simulink model "level3_MMC"  (Simulink 9.0)
settings: Solver=VariableStepAuto  StartTime=0.0  StopTime=10.0  RelTol=1e-3
libraries: powerlib x60
settings Model: Creator=lenovo  LastModifiedBy=lenovo
settings DataIOCC: SaveFormat=Dataset
settings OptimizationCC: LifeSpan=auto
settings DebuggingCC: UnderspecifiedInitializationDetection=Simplified  MergeDetectMultiDrivingBlocksExec=error  SFUnexpectedBacktrackingDiag=error  SFNoUnconditionalDefaultTransitionDiag=error  SFExecutionAtInitializationDiag=warning
settings HardwareCC: ProdBitPerPointer=64  ProdBitPerSizeT=64  ProdBitPerPtrDiffT=64  ProdLargestAtomicFloat=Float  ProdIntDivRoundTo=Zero  ProdEndianess=LittleEndian  ProdWordSize=64  ProdHWDeviceType=Intel->x86-64 (Windows64)
settings ModelReferenceCC: PropagateSignalLabelsOutOfModel=on
settings CodeAppCC: StateflowObjectComments=off
settings GRTTargetCC: TargetLangStandard=C99 (ISO)
settings ConfigComp: CovMetricSettings=dwe  CovHtmlReporting=off  CovSaveCumulativeToWorkspaceVar=off  CovSaveSingleToWorkspaceVar=off  CovExternalEMLEnable=on

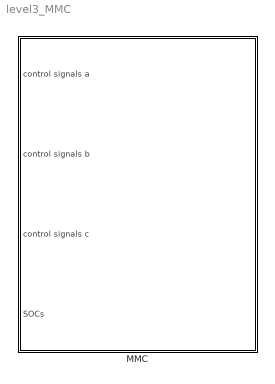
== system level3_MMC ==
  MMC : Subsystem

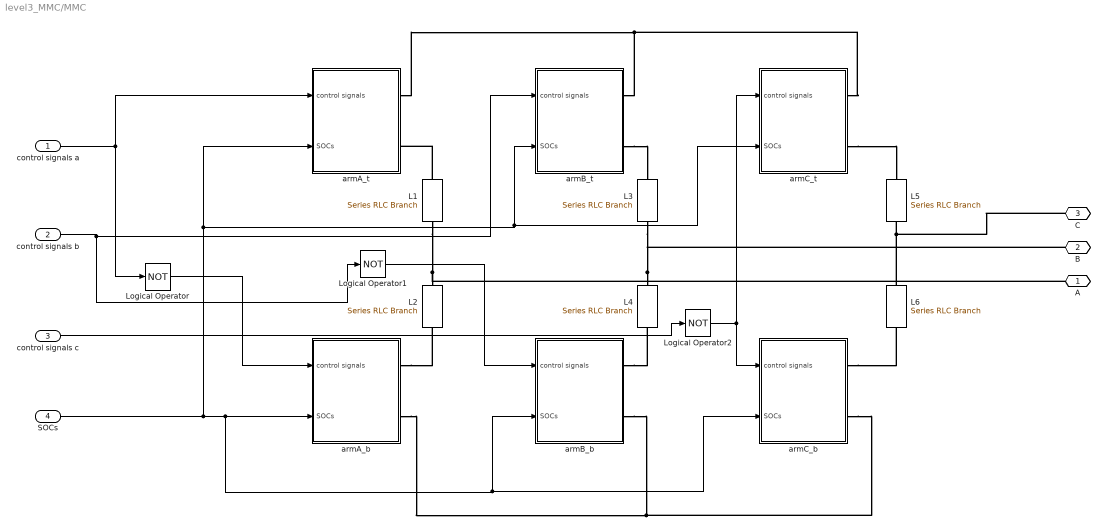
== system level3_MMC/MMC ==
  control signals a : Inport
  control signals b : Inport  Port=2
  control signals c : Inport  Port=3
  SOCs : Inport  Port=4
  L{1..6} (6 alike) : powerlib/Elements/Series RLC Branch  LConnTagsString=__new0  RConnTagsString=__new0  BranchType=L  Resistance=0  Inductance=50e-6  SetiL0=off  InitialCurrent=0  Capacitance=0  Setx0=off  InitialVoltage=0  Measurements=None
  Logical Operator : Logic  Operator=NOT  AllPortsSameDT=off  OutDataTypeStr=boolean
  Logical Operator1 : Logic  Operator=NOT  AllPortsSameDT=off  OutDataTypeStr=boolean
  Logical Operator2 : Logic  Operator=NOT  AllPortsSameDT=off  OutDataTypeStr=boolean
  armA_b : Subsystem
  armA_t : Subsystem
  armB_b : Subsystem
  armB_t : Subsystem
  armC_b : Subsystem
  armC_t : Subsystem
  A : PMIOPort  Port=1  Side=Right
  B : PMIOPort  Port=2  Side=Right
  C : PMIOPort  Port=3  Side=Right
  wires:
  SOCs/1 -> armA_b/2(SOCs), armC_b/2(SOCs), armB_b/2(SOCs), armA_t/2(SOCs), armC_t/2(SOCs), armB_t/2(SOCs)
  Logical Operator1/1 -> armB_b/1(control signals)
  control signals b/1 -> armB_t/1(control signals), Logical Operator1/1
  Logical Operator/1 -> armA_b/1(control signals)
  control signals a/1 -> armA_t/1(control signals), Logical Operator/1
  Logical Operator2/1 -> armC_b/1(control signals), armC_t/1(control signals)
  control signals c/1 -> Logical Operator2/1
  connections:
  L6/LConn1 -- C/RConn1 -- L5/RConn1
  L1/LConn1 -- armA_t/RConn2
  armC_t/RConn2 -- L5/LConn1
  armC_b/RConn1 -- L6/RConn1
  armB_t/RConn2 -- L3/LConn1
  armB_b/RConn1 -- L4/RConn1
  armA_b/RConn1 -- L2/RConn1
  L4/LConn1 -- L3/RConn1 -- B/RConn1
  L1/RConn1 -- L2/LConn1 -- A/RConn1
  armA_b/RConn2 -- armC_b/RConn2 -- armB_b/RConn2
  armA_t/RConn1 -- armC_t/RConn1 -- armB_t/RConn1

== system level3_MMC/MMC/armA_b ==
  control signals : Inport
  SOCs : Inport  Port=2
  SubModule1 : Subsystem
  SubModule2 : Subsystem
  SubModule3 : Subsystem
  Conn1 : PMIOPort  Port=1  Side=Right
  Conn2 : PMIOPort  Port=2  Side=Right
  wires:
  control signals/1 -> SubModule3/1(control signal), SubModule2/1(control signal), SubModule1/1(control signal)
  SOCs/1 -> SubModule3/2(SOC), SubModule2/2(SOC), SubModule1/2(SOC)
  connections:
  SubModule1/RConn2 -- SubModule2/RConn1
  SubModule1/RConn1 -- Conn1/RConn1
  Conn2/RConn1 -- SubModule3/RConn2
  SubModule2/RConn2 -- SubModule3/RConn1

== system level3_MMC/MMC/armA_t ==
  control signals : Inport
  SOCs : Inport  Port=2
  SubModule1 : Subsystem
  SubModule2 : Subsystem
  SubModule3 : Subsystem
  Conn1 : PMIOPort  Port=1  Side=Right
  Conn2 : PMIOPort  Port=2  Side=Right
  wires:
  control signals/1 -> SubModule3/1(control signal), SubModule2/1(control signal), SubModule1/1(control signal)
  SOCs/1 -> SubModule3/2(SOC), SubModule2/2(SOC), SubModule1/2(SOC)
  connections:
  SubModule1/RConn2 -- SubModule2/RConn1
  SubModule1/RConn1 -- Conn1/RConn1
  Conn2/RConn1 -- SubModule3/RConn2
  SubModule2/RConn2 -- SubModule3/RConn1

== system level3_MMC/MMC/armB_b ==
  control signals : Inport
  SOCs : Inport  Port=2
  SubModule1 : Subsystem
  SubModule2 : Subsystem
  SubModule3 : Subsystem
  Conn1 : PMIOPort  Port=1  Side=Right
  Conn2 : PMIOPort  Port=2  Side=Right
  wires:
  control signals/1 -> SubModule3/1(control signal), SubModule2/1(control signal), SubModule1/1(control signal)
  SOCs/1 -> SubModule3/2(SOC), SubModule2/2(SOC), SubModule1/2(SOC)
  connections:
  SubModule1/RConn2 -- SubModule2/RConn1
  SubModule1/RConn1 -- Conn1/RConn1
  Conn2/RConn1 -- SubModule3/RConn2
  SubModule2/RConn2 -- SubModule3/RConn1

== system level3_MMC/MMC/armB_t ==
  control signals : Inport
  SOCs : Inport  Port=2
  SubModule1 : Subsystem
  SubModule2 : Subsystem
  SubModule3 : Subsystem
  Conn1 : PMIOPort  Port=1  Side=Right
  Conn2 : PMIOPort  Port=2  Side=Right
  wires:
  control signals/1 -> SubModule3/1(control signal), SubModule2/1(control signal), SubModule1/1(control signal)
  SOCs/1 -> SubModule3/2(SOC), SubModule2/2(SOC), SubModule1/2(SOC)
  connections:
  SubModule1/RConn2 -- SubModule2/RConn1
  SubModule1/RConn1 -- Conn1/RConn1
  Conn2/RConn1 -- SubModule3/RConn2
  SubModule2/RConn2 -- SubModule3/RConn1

== system level3_MMC/MMC/armC_b ==
  control signals : Inport
  SOCs : Inport  Port=2
  SubModule1 : Subsystem
  SubModule2 : Subsystem
  SubModule3 : Subsystem
  Conn1 : PMIOPort  Port=1  Side=Right
  Conn2 : PMIOPort  Port=2  Side=Right
  wires:
  control signals/1 -> SubModule3/1(control signal), SubModule2/1(control signal), SubModule1/1(control signal)
  SOCs/1 -> SubModule3/2(SOC), SubModule2/2(SOC), SubModule1/2(SOC)
  connections:
  SubModule1/RConn2 -- SubModule2/RConn1
  SubModule1/RConn1 -- Conn1/RConn1
  Conn2/RConn1 -- SubModule3/RConn2
  SubModule2/RConn2 -- SubModule3/RConn1

== system level3_MMC/MMC/armC_t ==
  control signals : Inport
  SOCs : Inport  Port=2
  SubModule1 : Subsystem
  SubModule2 : Subsystem
  SubModule3 : Subsystem
  Conn1 : PMIOPort  Port=1  Side=Right
  Conn2 : PMIOPort  Port=2  Side=Right
  wires:
  control signals/1 -> SubModule3/1(control signal), SubModule2/1(control signal), SubModule1/1(control signal)
  SOCs/1 -> SubModule3/2(SOC), SubModule2/2(SOC), SubModule1/2(SOC)
  connections:
  SubModule1/RConn2 -- SubModule2/RConn1
  SubModule1/RConn1 -- Conn1/RConn1
  Conn2/RConn1 -- SubModule3/RConn2
  SubModule2/RConn2 -- SubModule3/RConn1

== system level3_MMC/MMC/armA_b/SubModule1 ==
  control signal : Inport
  SOC : Inport  Port=2
  MOSFET : Subsystem
  cell voltage : Subsystem
  P1 : PMIOPort  Tag=PMCPort  Port=1  Side=Right
  P2 : PMIOPort  Tag=PMCPort  Port=2  Side=Right
  wires:
  control signal/1 -> MOSFET/1(control signal)
  cell voltage/1(V) -> MOSFET/2(V)
  SOC/1 -> cell voltage/1(SOC)
  connections:
  P1/RConn1 -- MOSFET/RConn1
  P2/RConn1 -- MOSFET/RConn2

== system level3_MMC/MMC/armA_b/SubModule2 ==
  control signal : Inport
  SOC : Inport  Port=2
  MOSFET : Subsystem
  cell voltage : Subsystem
  P1 : PMIOPort  Tag=PMCPort  Port=1  Side=Right
  P2 : PMIOPort  Tag=PMCPort  Port=2  Side=Right
  wires:
  control signal/1 -> MOSFET/1(control signal)
  cell voltage/1(V) -> MOSFET/2(V)
  SOC/1 -> cell voltage/1(SOC)
  connections:
  P1/RConn1 -- MOSFET/RConn1
  P2/RConn1 -- MOSFET/RConn2

== system level3_MMC/MMC/armA_b/SubModule3 ==
  control signal : Inport
  SOC : Inport  Port=2
  MOSFET : Subsystem
  cell voltage : Subsystem
  P1 : PMIOPort  Tag=PMCPort  Port=1  Side=Right
  P2 : PMIOPort  Tag=PMCPort  Port=2  Side=Right
  wires:
  control signal/1 -> MOSFET/1(control signal)
  cell voltage/1(V) -> MOSFET/2(V)
  SOC/1 -> cell voltage/1(SOC)
  connections:
  P1/RConn1 -- MOSFET/RConn1
  P2/RConn1 -- MOSFET/RConn2

== system level3_MMC/MMC/armA_t/SubModule1 ==
  control signal : Inport
  SOC : Inport  Port=2
  MOSFET : Subsystem
  cell voltage : Subsystem
  P1 : PMIOPort  Tag=PMCPort  Port=1  Side=Right
  P2 : PMIOPort  Tag=PMCPort  Port=2  Side=Right
  wires:
  control signal/1 -> MOSFET/1(control signal)
  cell voltage/1(V) -> MOSFET/2(V)
  SOC/1 -> cell voltage/1(SOC)
  connections:
  P1/RConn1 -- MOSFET/RConn1
  P2/RConn1 -- MOSFET/RConn2

== system level3_MMC/MMC/armA_t/SubModule2 ==
  control signal : Inport
  SOC : Inport  Port=2
  MOSFET : Subsystem
  cell voltage : Subsystem
  P1 : PMIOPort  Tag=PMCPort  Port=1  Side=Right
  P2 : PMIOPort  Tag=PMCPort  Port=2  Side=Right
  wires:
  control signal/1 -> MOSFET/1(control signal)
  cell voltage/1(V) -> MOSFET/2(V)
  SOC/1 -> cell voltage/1(SOC)
  connections:
  P1/RConn1 -- MOSFET/RConn1
  P2/RConn1 -- MOSFET/RConn2

== system level3_MMC/MMC/armA_t/SubModule3 ==
  control signal : Inport
  SOC : Inport  Port=2
  MOSFET : Subsystem
  cell voltage : Subsystem
  P1 : PMIOPort  Tag=PMCPort  Port=1  Side=Right
  P2 : PMIOPort  Tag=PMCPort  Port=2  Side=Right
  wires:
  control signal/1 -> MOSFET/1(control signal)
  cell voltage/1(V) -> MOSFET/2(V)
  SOC/1 -> cell voltage/1(SOC)
  connections:
  P1/RConn1 -- MOSFET/RConn1
  P2/RConn1 -- MOSFET/RConn2

== system level3_MMC/MMC/armB_b/SubModule1 ==
  control signal : Inport
  SOC : Inport  Port=2
  MOSFET : Subsystem
  cell voltage : Subsystem
  P1 : PMIOPort  Tag=PMCPort  Port=1  Side=Right
  P2 : PMIOPort  Tag=PMCPort  Port=2  Side=Right
  wires:
  control signal/1 -> MOSFET/1(control signal)
  cell voltage/1(V) -> MOSFET/2(V)
  SOC/1 -> cell voltage/1(SOC)
  connections:
  P1/RConn1 -- MOSFET/RConn1
  P2/RConn1 -- MOSFET/RConn2

== system level3_MMC/MMC/armB_b/SubModule2 ==
  control signal : Inport
  SOC : Inport  Port=2
  MOSFET : Subsystem
  cell voltage : Subsystem
  P1 : PMIOPort  Tag=PMCPort  Port=1  Side=Right
  P2 : PMIOPort  Tag=PMCPort  Port=2  Side=Right
  wires:
  control signal/1 -> MOSFET/1(control signal)
  cell voltage/1(V) -> MOSFET/2(V)
  SOC/1 -> cell voltage/1(SOC)
  connections:
  P1/RConn1 -- MOSFET/RConn1
  P2/RConn1 -- MOSFET/RConn2

== system level3_MMC/MMC/armB_b/SubModule3 ==
  control signal : Inport
  SOC : Inport  Port=2
  MOSFET : Subsystem
  cell voltage : Subsystem
  P1 : PMIOPort  Tag=PMCPort  Port=1  Side=Right
  P2 : PMIOPort  Tag=PMCPort  Port=2  Side=Right
  wires:
  control signal/1 -> MOSFET/1(control signal)
  cell voltage/1(V) -> MOSFET/2(V)
  SOC/1 -> cell voltage/1(SOC)
  connections:
  P1/RConn1 -- MOSFET/RConn1
  P2/RConn1 -- MOSFET/RConn2

== system level3_MMC/MMC/armB_t/SubModule1 ==
  control signal : Inport
  SOC : Inport  Port=2
  MOSFET : Subsystem
  cell voltage : Subsystem
  P1 : PMIOPort  Tag=PMCPort  Port=1  Side=Right
  P2 : PMIOPort  Tag=PMCPort  Port=2  Side=Right
  wires:
  control signal/1 -> MOSFET/1(control signal)
  cell voltage/1(V) -> MOSFET/2(V)
  SOC/1 -> cell voltage/1(SOC)
  connections:
  P1/RConn1 -- MOSFET/RConn1
  P2/RConn1 -- MOSFET/RConn2

== system level3_MMC/MMC/armB_t/SubModule2 ==
  control signal : Inport
  SOC : Inport  Port=2
  MOSFET : Subsystem
  cell voltage : Subsystem
  P1 : PMIOPort  Tag=PMCPort  Port=1  Side=Right
  P2 : PMIOPort  Tag=PMCPort  Port=2  Side=Right
  wires:
  control signal/1 -> MOSFET/1(control signal)
  cell voltage/1(V) -> MOSFET/2(V)
  SOC/1 -> cell voltage/1(SOC)
  connections:
  P1/RConn1 -- MOSFET/RConn1
  P2/RConn1 -- MOSFET/RConn2

== system level3_MMC/MMC/armB_t/SubModule3 ==
  control signal : Inport
  SOC : Inport  Port=2
  MOSFET : Subsystem
  cell voltage : Subsystem
  P1 : PMIOPort  Tag=PMCPort  Port=1  Side=Right
  P2 : PMIOPort  Tag=PMCPort  Port=2  Side=Right
  wires:
  control signal/1 -> MOSFET/1(control signal)
  cell voltage/1(V) -> MOSFET/2(V)
  SOC/1 -> cell voltage/1(SOC)
  connections:
  P1/RConn1 -- MOSFET/RConn1
  P2/RConn1 -- MOSFET/RConn2

== system level3_MMC/MMC/armC_b/SubModule1 ==
  control signal : Inport
  SOC : Inport  Port=2
  MOSFET : Subsystem
  cell voltage : Subsystem
  P1 : PMIOPort  Tag=PMCPort  Port=1  Side=Right
  P2 : PMIOPort  Tag=PMCPort  Port=2  Side=Right
  wires:
  control signal/1 -> MOSFET/1(control signal)
  cell voltage/1(V) -> MOSFET/2(V)
  SOC/1 -> cell voltage/1(SOC)
  connections:
  P1/RConn1 -- MOSFET/RConn1
  P2/RConn1 -- MOSFET/RConn2

== system level3_MMC/MMC/armC_b/SubModule2 ==
  control signal : Inport
  SOC : Inport  Port=2
  MOSFET : Subsystem
  cell voltage : Subsystem
  P1 : PMIOPort  Tag=PMCPort  Port=1  Side=Right
  P2 : PMIOPort  Tag=PMCPort  Port=2  Side=Right
  wires:
  control signal/1 -> MOSFET/1(control signal)
  cell voltage/1(V) -> MOSFET/2(V)
  SOC/1 -> cell voltage/1(SOC)
  connections:
  P1/RConn1 -- MOSFET/RConn1
  P2/RConn1 -- MOSFET/RConn2

== system level3_MMC/MMC/armC_b/SubModule3 ==
  control signal : Inport
  SOC : Inport  Port=2
  MOSFET : Subsystem
  cell voltage : Subsystem
  P1 : PMIOPort  Tag=PMCPort  Port=1  Side=Right
  P2 : PMIOPort  Tag=PMCPort  Port=2  Side=Right
  wires:
  control signal/1 -> MOSFET/1(control signal)
  cell voltage/1(V) -> MOSFET/2(V)
  SOC/1 -> cell voltage/1(SOC)
  connections:
  P1/RConn1 -- MOSFET/RConn1
  P2/RConn1 -- MOSFET/RConn2

== system level3_MMC/MMC/armC_t/SubModule1 ==
  control signal : Inport
  SOC : Inport  Port=2
  MOSFET : Subsystem
  cell voltage : Subsystem
  P1 : PMIOPort  Tag=PMCPort  Port=1  Side=Right
  P2 : PMIOPort  Tag=PMCPort  Port=2  Side=Right
  wires:
  control signal/1 -> MOSFET/1(control signal)
  cell voltage/1(V) -> MOSFET/2(V)
  SOC/1 -> cell voltage/1(SOC)
  connections:
  P1/RConn1 -- MOSFET/RConn1
  P2/RConn1 -- MOSFET/RConn2

== system level3_MMC/MMC/armC_t/SubModule2 ==
  control signal : Inport
  SOC : Inport  Port=2
  MOSFET : Subsystem
  cell voltage : Subsystem
  P1 : PMIOPort  Tag=PMCPort  Port=1  Side=Right
  P2 : PMIOPort  Tag=PMCPort  Port=2  Side=Right
  wires:
  control signal/1 -> MOSFET/1(control signal)
  cell voltage/1(V) -> MOSFET/2(V)
  SOC/1 -> cell voltage/1(SOC)
  connections:
  P1/RConn1 -- MOSFET/RConn1
  P2/RConn1 -- MOSFET/RConn2

== system level3_MMC/MMC/armC_t/SubModule3 ==
  control signal : Inport
  SOC : Inport  Port=2
  MOSFET : Subsystem
  cell voltage : Subsystem
  P1 : PMIOPort  Tag=PMCPort  Port=1  Side=Right
  P2 : PMIOPort  Tag=PMCPort  Port=2  Side=Right
  wires:
  control signal/1 -> MOSFET/1(control signal)
  cell voltage/1(V) -> MOSFET/2(V)
  SOC/1 -> cell voltage/1(SOC)
  connections:
  P1/RConn1 -- MOSFET/RConn1
  P2/RConn1 -- MOSFET/RConn2

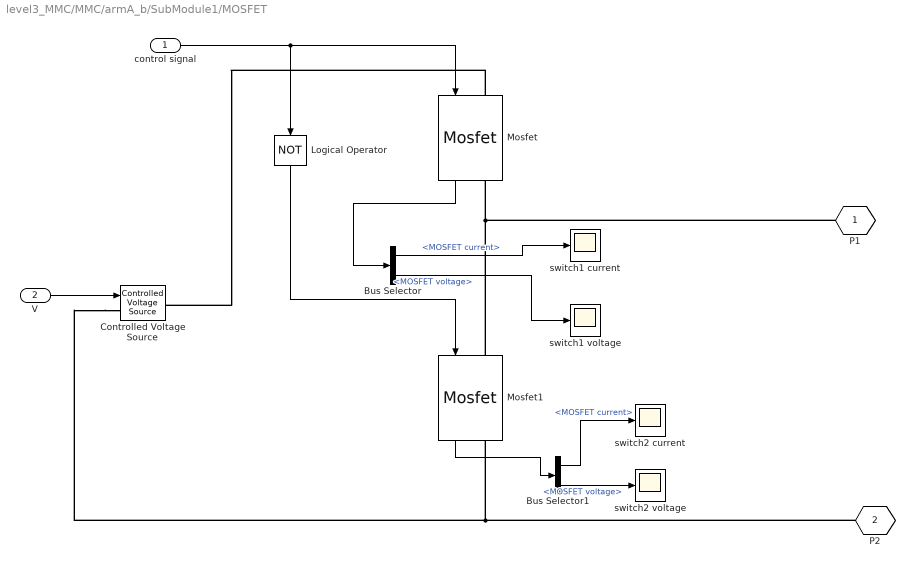
== system level3_MMC/MMC/armA_b/SubModule1/MOSFET ==
  control signal : Inport
  V : Inport  Port=2
  Bus Selector : BusSelector  OutputSignals=MOSFET current,MOSFET voltage
  Bus Selector1 : BusSelector  OutputSignals=MOSFET current,MOSFET voltage
  Controlled Voltage Source : powerlib/Electrical Sources/Controlled Voltage Source  Initialize=on  Source_Type=AC  Amplitude=0  Phase=0  Frequency=0  Measurements=None
  Logical Operator : Logic  Operator=NOT  AllPortsSameDT=off  OutDataTypeStr=boolean
  Mosfet : powerlib/Power Electronics/Mosfet  Ron=0.0005  Lon=0  Rd=0.01  Vfd=0  IC=0  Rs=1e5  Cs=inf  Measurements=on
  Mosfet1 : powerlib/Power Electronics/Mosfet  Ron=0.0005  Lon=0  Rd=0.01  Vfd=0  IC=0  Rs=1e5  Cs=inf  Measurements=on
  switch1 current : Scope
  switch1 voltage : Scope
  switch2 current : Scope
  switch2 voltage : Scope
  P1 : PMIOPort  Tag=PMCPort  Port=1  Side=Right
  P2 : PMIOPort  Tag=PMCPort  Port=2  Side=Right
  wires:
  control signal/1 -> Logical Operator/1, Mosfet/1
  Mosfet/1 -> Bus Selector/1
  V/1 -> Controlled Voltage Source/1
  Bus Selector/1 -> switch1 current/1  "<MOSFET current>"
  Bus Selector/2 -> switch1 voltage/1  "<MOSFET voltage>"
  Bus Selector1/1 -> switch2 current/1  "<MOSFET current>"
  Bus Selector1/2 -> switch2 voltage/1  "<MOSFET voltage>"
  Logical Operator/1 -> Mosfet1/1
  Mosfet1/1 -> Bus Selector1/1
  connections:
  Controlled Voltage Source/LConn1 -- Mosfet1/RConn1 -- P2/RConn1
  Mosfet1/LConn1 -- Mosfet/RConn1 -- P1/RConn1
  Mosfet/LConn1 -- Controlled Voltage Source/RConn1

== system level3_MMC/MMC/armA_b/SubModule1/cell voltage ==
  SOC : Inport
  Constant : Constant  Value=3
  Gain : Gain  Gain=1.2
  Sum : Sum  Inputs=|++
  V : Outport
  wires:
  Sum/1 -> V/1
  SOC/1 -> Gain/1
  Gain/1 -> Sum/2
  Constant/1 -> Sum/1

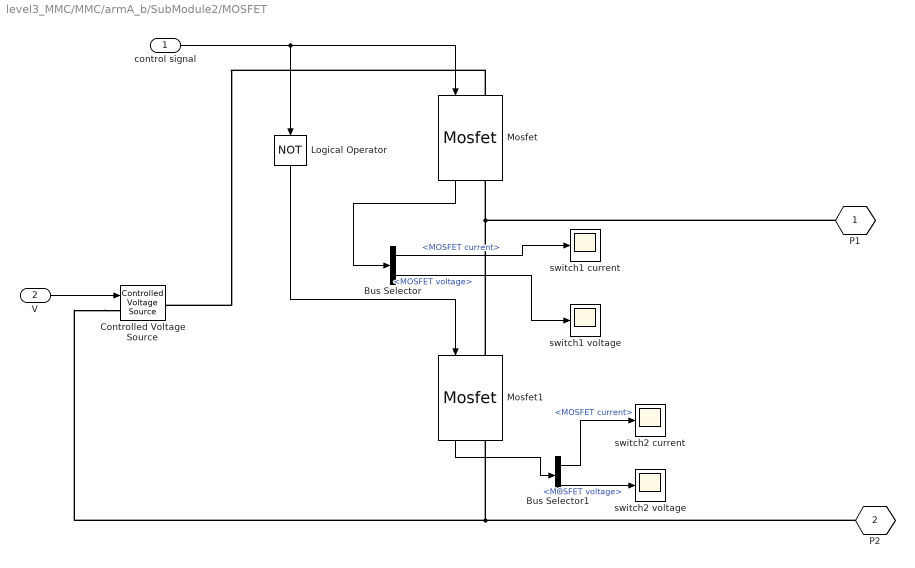
== system level3_MMC/MMC/armA_b/SubModule2/MOSFET ==
  control signal : Inport
  V : Inport  Port=2
  Bus Selector : BusSelector  OutputSignals=MOSFET current,MOSFET voltage
  Bus Selector1 : BusSelector  OutputSignals=MOSFET current,MOSFET voltage
  Controlled Voltage Source : powerlib/Electrical Sources/Controlled Voltage Source  Initialize=on  Source_Type=AC  Amplitude=0  Phase=0  Frequency=0  Measurements=None
  Logical Operator : Logic  Operator=NOT  AllPortsSameDT=off  OutDataTypeStr=boolean
  Mosfet : powerlib/Power Electronics/Mosfet  Ron=0.0005  Lon=0  Rd=0.01  Vfd=0  IC=0  Rs=1e5  Cs=inf  Measurements=on
  Mosfet1 : powerlib/Power Electronics/Mosfet  Ron=0.0005  Lon=0  Rd=0.01  Vfd=0  IC=0  Rs=1e5  Cs=inf  Measurements=on
  switch1 current : Scope
  switch1 voltage : Scope
  switch2 current : Scope
  switch2 voltage : Scope
  P1 : PMIOPort  Tag=PMCPort  Port=1  Side=Right
  P2 : PMIOPort  Tag=PMCPort  Port=2  Side=Right
  wires:
  control signal/1 -> Logical Operator/1, Mosfet/1
  Mosfet/1 -> Bus Selector/1
  V/1 -> Controlled Voltage Source/1
  Bus Selector/1 -> switch1 current/1  "<MOSFET current>"
  Bus Selector/2 -> switch1 voltage/1  "<MOSFET voltage>"
  Bus Selector1/1 -> switch2 current/1  "<MOSFET current>"
  Bus Selector1/2 -> switch2 voltage/1  "<MOSFET voltage>"
  Logical Operator/1 -> Mosfet1/1
  Mosfet1/1 -> Bus Selector1/1
  connections:
  Controlled Voltage Source/LConn1 -- Mosfet1/RConn1 -- P2/RConn1
  Mosfet1/LConn1 -- Mosfet/RConn1 -- P1/RConn1
  Mosfet/LConn1 -- Controlled Voltage Source/RConn1

== system level3_MMC/MMC/armA_b/SubModule2/cell voltage ==
  SOC : Inport
  Constant : Constant  Value=3
  Gain : Gain  Gain=1.2
  Sum : Sum  Inputs=|++
  V : Outport
  wires:
  Sum/1 -> V/1
  SOC/1 -> Gain/1
  Gain/1 -> Sum/2
  Constant/1 -> Sum/1

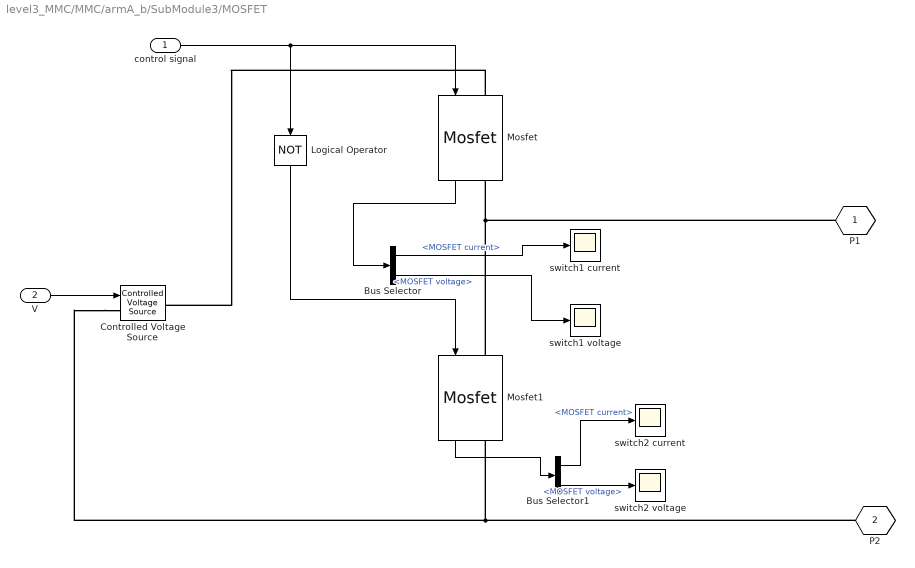
== system level3_MMC/MMC/armA_b/SubModule3/MOSFET ==
  control signal : Inport
  V : Inport  Port=2
  Bus Selector : BusSelector  OutputSignals=MOSFET current,MOSFET voltage
  Bus Selector1 : BusSelector  OutputSignals=MOSFET current,MOSFET voltage
  Controlled Voltage Source : powerlib/Electrical Sources/Controlled Voltage Source  Initialize=on  Source_Type=AC  Amplitude=0  Phase=0  Frequency=0  Measurements=None
  Logical Operator : Logic  Operator=NOT  AllPortsSameDT=off  OutDataTypeStr=boolean
  Mosfet : powerlib/Power Electronics/Mosfet  Ron=0.0005  Lon=0  Rd=0.01  Vfd=0  IC=0  Rs=1e5  Cs=inf  Measurements=on
  Mosfet1 : powerlib/Power Electronics/Mosfet  Ron=0.0005  Lon=0  Rd=0.01  Vfd=0  IC=0  Rs=1e5  Cs=inf  Measurements=on
  switch1 current : Scope
  switch1 voltage : Scope
  switch2 current : Scope
  switch2 voltage : Scope
  P1 : PMIOPort  Tag=PMCPort  Port=1  Side=Right
  P2 : PMIOPort  Tag=PMCPort  Port=2  Side=Right
  wires:
  control signal/1 -> Logical Operator/1, Mosfet/1
  Mosfet/1 -> Bus Selector/1
  V/1 -> Controlled Voltage Source/1
  Bus Selector/1 -> switch1 current/1  "<MOSFET current>"
  Bus Selector/2 -> switch1 voltage/1  "<MOSFET voltage>"
  Bus Selector1/1 -> switch2 current/1  "<MOSFET current>"
  Bus Selector1/2 -> switch2 voltage/1  "<MOSFET voltage>"
  Logical Operator/1 -> Mosfet1/1
  Mosfet1/1 -> Bus Selector1/1
  connections:
  Controlled Voltage Source/LConn1 -- Mosfet1/RConn1 -- P2/RConn1
  Mosfet1/LConn1 -- Mosfet/RConn1 -- P1/RConn1
  Mosfet/LConn1 -- Controlled Voltage Source/RConn1

== system level3_MMC/MMC/armA_b/SubModule3/cell voltage ==
  SOC : Inport
  Constant : Constant  Value=3
  Gain : Gain  Gain=1.2
  Sum : Sum  Inputs=|++
  V : Outport
  wires:
  Sum/1 -> V/1
  SOC/1 -> Gain/1
  Gain/1 -> Sum/2
  Constant/1 -> Sum/1

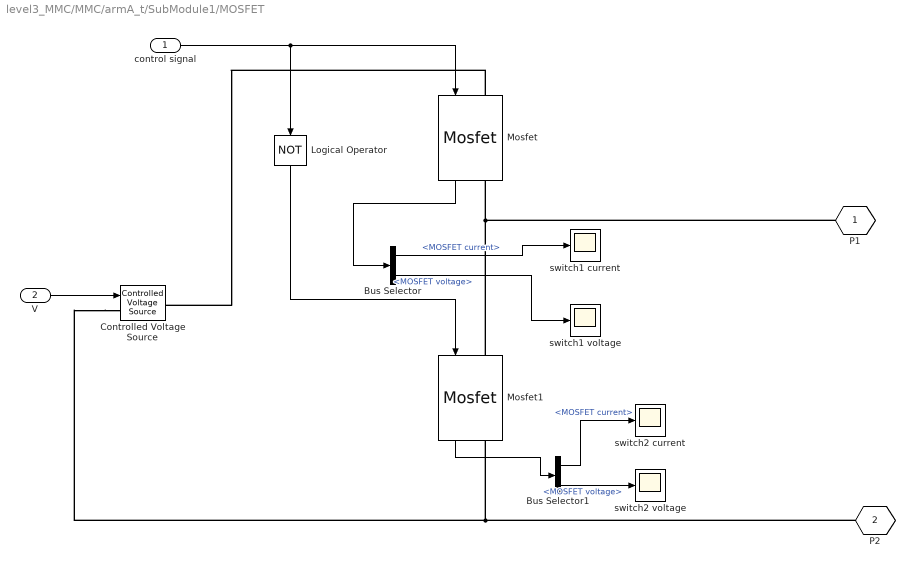
== system level3_MMC/MMC/armA_t/SubModule1/MOSFET ==
  control signal : Inport
  V : Inport  Port=2
  Bus Selector : BusSelector  OutputSignals=MOSFET current,MOSFET voltage
  Bus Selector1 : BusSelector  OutputSignals=MOSFET current,MOSFET voltage
  Controlled Voltage Source : powerlib/Electrical Sources/Controlled Voltage Source  Initialize=on  Source_Type=AC  Amplitude=0  Phase=0  Frequency=0  Measurements=None
  Logical Operator : Logic  Operator=NOT  AllPortsSameDT=off  OutDataTypeStr=boolean
  Mosfet : powerlib/Power Electronics/Mosfet  Ron=0.0005  Lon=0  Rd=0.01  Vfd=0  IC=0  Rs=1e5  Cs=inf  Measurements=on
  Mosfet1 : powerlib/Power Electronics/Mosfet  Ron=0.0005  Lon=0  Rd=0.01  Vfd=0  IC=0  Rs=1e5  Cs=inf  Measurements=on
  switch1 current : Scope
  switch1 voltage : Scope
  switch2 current : Scope
  switch2 voltage : Scope
  P1 : PMIOPort  Tag=PMCPort  Port=1  Side=Right
  P2 : PMIOPort  Tag=PMCPort  Port=2  Side=Right
  wires:
  control signal/1 -> Logical Operator/1, Mosfet/1
  Mosfet/1 -> Bus Selector/1
  V/1 -> Controlled Voltage Source/1
  Bus Selector/1 -> switch1 current/1  "<MOSFET current>"
  Bus Selector/2 -> switch1 voltage/1  "<MOSFET voltage>"
  Bus Selector1/1 -> switch2 current/1  "<MOSFET current>"
  Bus Selector1/2 -> switch2 voltage/1  "<MOSFET voltage>"
  Logical Operator/1 -> Mosfet1/1
  Mosfet1/1 -> Bus Selector1/1
  connections:
  Controlled Voltage Source/LConn1 -- Mosfet1/RConn1 -- P2/RConn1
  Mosfet1/LConn1 -- Mosfet/RConn1 -- P1/RConn1
  Mosfet/LConn1 -- Controlled Voltage Source/RConn1

== system level3_MMC/MMC/armA_t/SubModule1/cell voltage ==
  SOC : Inport
  Constant : Constant  Value=3
  Gain : Gain  Gain=1.2
  Sum : Sum  Inputs=|++
  V : Outport
  wires:
  Sum/1 -> V/1
  SOC/1 -> Gain/1
  Gain/1 -> Sum/2
  Constant/1 -> Sum/1

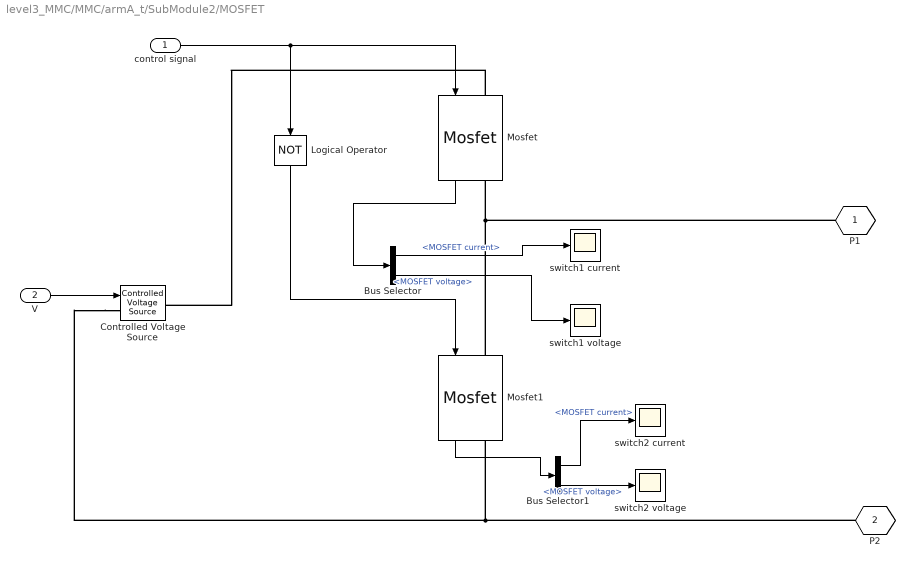
== system level3_MMC/MMC/armA_t/SubModule2/MOSFET ==
  control signal : Inport
  V : Inport  Port=2
  Bus Selector : BusSelector  OutputSignals=MOSFET current,MOSFET voltage
  Bus Selector1 : BusSelector  OutputSignals=MOSFET current,MOSFET voltage
  Controlled Voltage Source : powerlib/Electrical Sources/Controlled Voltage Source  Initialize=on  Source_Type=AC  Amplitude=0  Phase=0  Frequency=0  Measurements=None
  Logical Operator : Logic  Operator=NOT  AllPortsSameDT=off  OutDataTypeStr=boolean
  Mosfet : powerlib/Power Electronics/Mosfet  Ron=0.0005  Lon=0  Rd=0.01  Vfd=0  IC=0  Rs=1e5  Cs=inf  Measurements=on
  Mosfet1 : powerlib/Power Electronics/Mosfet  Ron=0.0005  Lon=0  Rd=0.01  Vfd=0  IC=0  Rs=1e5  Cs=inf  Measurements=on
  switch1 current : Scope
  switch1 voltage : Scope
  switch2 current : Scope
  switch2 voltage : Scope
  P1 : PMIOPort  Tag=PMCPort  Port=1  Side=Right
  P2 : PMIOPort  Tag=PMCPort  Port=2  Side=Right
  wires:
  control signal/1 -> Logical Operator/1, Mosfet/1
  Mosfet/1 -> Bus Selector/1
  V/1 -> Controlled Voltage Source/1
  Bus Selector/1 -> switch1 current/1  "<MOSFET current>"
  Bus Selector/2 -> switch1 voltage/1  "<MOSFET voltage>"
  Bus Selector1/1 -> switch2 current/1  "<MOSFET current>"
  Bus Selector1/2 -> switch2 voltage/1  "<MOSFET voltage>"
  Logical Operator/1 -> Mosfet1/1
  Mosfet1/1 -> Bus Selector1/1
  connections:
  Controlled Voltage Source/LConn1 -- Mosfet1/RConn1 -- P2/RConn1
  Mosfet1/LConn1 -- Mosfet/RConn1 -- P1/RConn1
  Mosfet/LConn1 -- Controlled Voltage Source/RConn1

== system level3_MMC/MMC/armA_t/SubModule2/cell voltage ==
  SOC : Inport
  Constant : Constant  Value=3
  Gain : Gain  Gain=1.2
  Sum : Sum  Inputs=|++
  V : Outport
  wires:
  Sum/1 -> V/1
  SOC/1 -> Gain/1
  Gain/1 -> Sum/2
  Constant/1 -> Sum/1

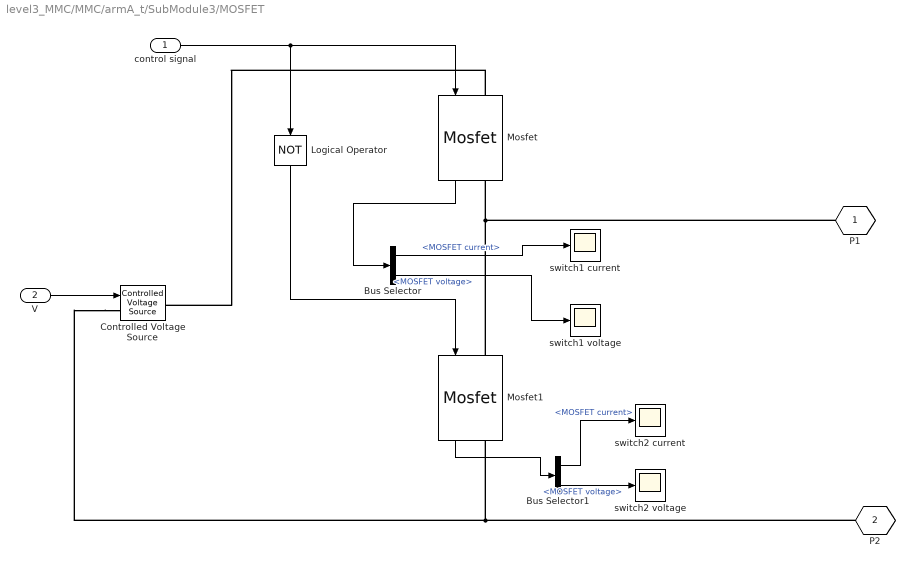
== system level3_MMC/MMC/armA_t/SubModule3/MOSFET ==
  control signal : Inport
  V : Inport  Port=2
  Bus Selector : BusSelector  OutputSignals=MOSFET current,MOSFET voltage
  Bus Selector1 : BusSelector  OutputSignals=MOSFET current,MOSFET voltage
  Controlled Voltage Source : powerlib/Electrical Sources/Controlled Voltage Source  Initialize=on  Source_Type=AC  Amplitude=0  Phase=0  Frequency=0  Measurements=None
  Logical Operator : Logic  Operator=NOT  AllPortsSameDT=off  OutDataTypeStr=boolean
  Mosfet : powerlib/Power Electronics/Mosfet  Ron=0.0005  Lon=0  Rd=0.01  Vfd=0  IC=0  Rs=1e5  Cs=inf  Measurements=on
  Mosfet1 : powerlib/Power Electronics/Mosfet  Ron=0.0005  Lon=0  Rd=0.01  Vfd=0  IC=0  Rs=1e5  Cs=inf  Measurements=on
  switch1 current : Scope
  switch1 voltage : Scope
  switch2 current : Scope
  switch2 voltage : Scope
  P1 : PMIOPort  Tag=PMCPort  Port=1  Side=Right
  P2 : PMIOPort  Tag=PMCPort  Port=2  Side=Right
  wires:
  control signal/1 -> Logical Operator/1, Mosfet/1
  Mosfet/1 -> Bus Selector/1
  V/1 -> Controlled Voltage Source/1
  Bus Selector/1 -> switch1 current/1  "<MOSFET current>"
  Bus Selector/2 -> switch1 voltage/1  "<MOSFET voltage>"
  Bus Selector1/1 -> switch2 current/1  "<MOSFET current>"
  Bus Selector1/2 -> switch2 voltage/1  "<MOSFET voltage>"
  Logical Operator/1 -> Mosfet1/1
  Mosfet1/1 -> Bus Selector1/1
  connections:
  Controlled Voltage Source/LConn1 -- Mosfet1/RConn1 -- P2/RConn1
  Mosfet1/LConn1 -- Mosfet/RConn1 -- P1/RConn1
  Mosfet/LConn1 -- Controlled Voltage Source/RConn1

== system level3_MMC/MMC/armA_t/SubModule3/cell voltage ==
  SOC : Inport
  Constant : Constant  Value=3
  Gain : Gain  Gain=1.2
  Sum : Sum  Inputs=|++
  V : Outport
  wires:
  Sum/1 -> V/1
  SOC/1 -> Gain/1
  Gain/1 -> Sum/2
  Constant/1 -> Sum/1

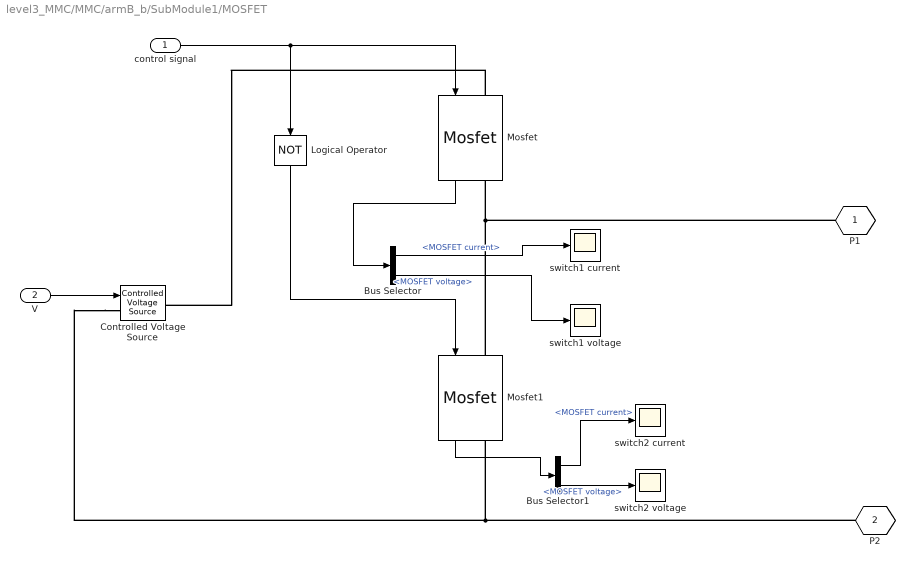
== system level3_MMC/MMC/armB_b/SubModule1/MOSFET ==
  control signal : Inport
  V : Inport  Port=2
  Bus Selector : BusSelector  OutputSignals=MOSFET current,MOSFET voltage
  Bus Selector1 : BusSelector  OutputSignals=MOSFET current,MOSFET voltage
  Controlled Voltage Source : powerlib/Electrical Sources/Controlled Voltage Source  Initialize=on  Source_Type=AC  Amplitude=0  Phase=0  Frequency=0  Measurements=None
  Logical Operator : Logic  Operator=NOT  AllPortsSameDT=off  OutDataTypeStr=boolean
  Mosfet : powerlib/Power Electronics/Mosfet  Ron=0.0005  Lon=0  Rd=0.01  Vfd=0  IC=0  Rs=1e5  Cs=inf  Measurements=on
  Mosfet1 : powerlib/Power Electronics/Mosfet  Ron=0.0005  Lon=0  Rd=0.01  Vfd=0  IC=0  Rs=1e5  Cs=inf  Measurements=on
  switch1 current : Scope
  switch1 voltage : Scope
  switch2 current : Scope
  switch2 voltage : Scope
  P1 : PMIOPort  Tag=PMCPort  Port=1  Side=Right
  P2 : PMIOPort  Tag=PMCPort  Port=2  Side=Right
  wires:
  control signal/1 -> Logical Operator/1, Mosfet/1
  Mosfet/1 -> Bus Selector/1
  V/1 -> Controlled Voltage Source/1
  Bus Selector/1 -> switch1 current/1  "<MOSFET current>"
  Bus Selector/2 -> switch1 voltage/1  "<MOSFET voltage>"
  Bus Selector1/1 -> switch2 current/1  "<MOSFET current>"
  Bus Selector1/2 -> switch2 voltage/1  "<MOSFET voltage>"
  Logical Operator/1 -> Mosfet1/1
  Mosfet1/1 -> Bus Selector1/1
  connections:
  Controlled Voltage Source/LConn1 -- Mosfet1/RConn1 -- P2/RConn1
  Mosfet1/LConn1 -- Mosfet/RConn1 -- P1/RConn1
  Mosfet/LConn1 -- Controlled Voltage Source/RConn1

== system level3_MMC/MMC/armB_b/SubModule1/cell voltage ==
  SOC : Inport
  Constant : Constant  Value=3
  Gain : Gain  Gain=1.2
  Sum : Sum  Inputs=|++
  V : Outport
  wires:
  Sum/1 -> V/1
  SOC/1 -> Gain/1
  Gain/1 -> Sum/2
  Constant/1 -> Sum/1

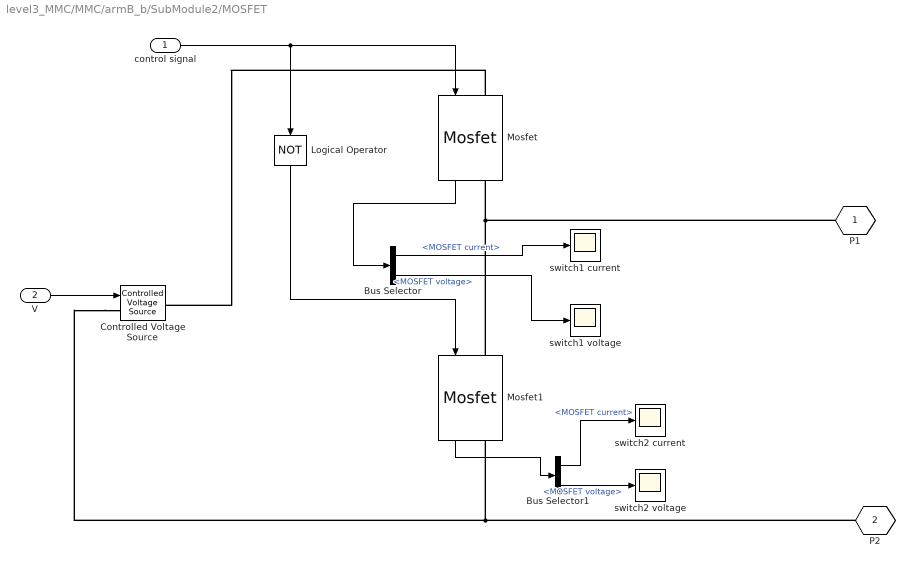
== system level3_MMC/MMC/armB_b/SubModule2/MOSFET ==
  control signal : Inport
  V : Inport  Port=2
  Bus Selector : BusSelector  OutputSignals=MOSFET current,MOSFET voltage
  Bus Selector1 : BusSelector  OutputSignals=MOSFET current,MOSFET voltage
  Controlled Voltage Source : powerlib/Electrical Sources/Controlled Voltage Source  Initialize=on  Source_Type=AC  Amplitude=0  Phase=0  Frequency=0  Measurements=None
  Logical Operator : Logic  Operator=NOT  AllPortsSameDT=off  OutDataTypeStr=boolean
  Mosfet : powerlib/Power Electronics/Mosfet  Ron=0.0005  Lon=0  Rd=0.01  Vfd=0  IC=0  Rs=1e5  Cs=inf  Measurements=on
  Mosfet1 : powerlib/Power Electronics/Mosfet  Ron=0.0005  Lon=0  Rd=0.01  Vfd=0  IC=0  Rs=1e5  Cs=inf  Measurements=on
  switch1 current : Scope
  switch1 voltage : Scope
  switch2 current : Scope
  switch2 voltage : Scope
  P1 : PMIOPort  Tag=PMCPort  Port=1  Side=Right
  P2 : PMIOPort  Tag=PMCPort  Port=2  Side=Right
  wires:
  control signal/1 -> Logical Operator/1, Mosfet/1
  Mosfet/1 -> Bus Selector/1
  V/1 -> Controlled Voltage Source/1
  Bus Selector/1 -> switch1 current/1  "<MOSFET current>"
  Bus Selector/2 -> switch1 voltage/1  "<MOSFET voltage>"
  Bus Selector1/1 -> switch2 current/1  "<MOSFET current>"
  Bus Selector1/2 -> switch2 voltage/1  "<MOSFET voltage>"
  Logical Operator/1 -> Mosfet1/1
  Mosfet1/1 -> Bus Selector1/1
  connections:
  Controlled Voltage Source/LConn1 -- Mosfet1/RConn1 -- P2/RConn1
  Mosfet1/LConn1 -- Mosfet/RConn1 -- P1/RConn1
  Mosfet/LConn1 -- Controlled Voltage Source/RConn1

== system level3_MMC/MMC/armB_b/SubModule2/cell voltage ==
  SOC : Inport
  Constant : Constant  Value=3
  Gain : Gain  Gain=1.2
  Sum : Sum  Inputs=|++
  V : Outport
  wires:
  Sum/1 -> V/1
  SOC/1 -> Gain/1
  Gain/1 -> Sum/2
  Constant/1 -> Sum/1

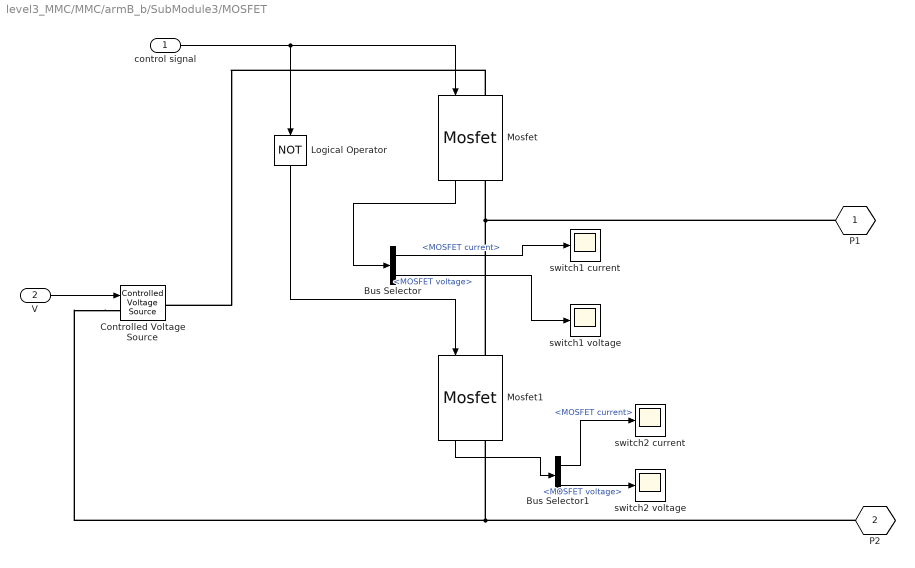
== system level3_MMC/MMC/armB_b/SubModule3/MOSFET ==
  control signal : Inport
  V : Inport  Port=2
  Bus Selector : BusSelector  OutputSignals=MOSFET current,MOSFET voltage
  Bus Selector1 : BusSelector  OutputSignals=MOSFET current,MOSFET voltage
  Controlled Voltage Source : powerlib/Electrical Sources/Controlled Voltage Source  Initialize=on  Source_Type=AC  Amplitude=0  Phase=0  Frequency=0  Measurements=None
  Logical Operator : Logic  Operator=NOT  AllPortsSameDT=off  OutDataTypeStr=boolean
  Mosfet : powerlib/Power Electronics/Mosfet  Ron=0.0005  Lon=0  Rd=0.01  Vfd=0  IC=0  Rs=1e5  Cs=inf  Measurements=on
  Mosfet1 : powerlib/Power Electronics/Mosfet  Ron=0.0005  Lon=0  Rd=0.01  Vfd=0  IC=0  Rs=1e5  Cs=inf  Measurements=on
  switch1 current : Scope
  switch1 voltage : Scope
  switch2 current : Scope
  switch2 voltage : Scope
  P1 : PMIOPort  Tag=PMCPort  Port=1  Side=Right
  P2 : PMIOPort  Tag=PMCPort  Port=2  Side=Right
  wires:
  control signal/1 -> Logical Operator/1, Mosfet/1
  Mosfet/1 -> Bus Selector/1
  V/1 -> Controlled Voltage Source/1
  Bus Selector/1 -> switch1 current/1  "<MOSFET current>"
  Bus Selector/2 -> switch1 voltage/1  "<MOSFET voltage>"
  Bus Selector1/1 -> switch2 current/1  "<MOSFET current>"
  Bus Selector1/2 -> switch2 voltage/1  "<MOSFET voltage>"
  Logical Operator/1 -> Mosfet1/1
  Mosfet1/1 -> Bus Selector1/1
  connections:
  Controlled Voltage Source/LConn1 -- Mosfet1/RConn1 -- P2/RConn1
  Mosfet1/LConn1 -- Mosfet/RConn1 -- P1/RConn1
  Mosfet/LConn1 -- Controlled Voltage Source/RConn1

== system level3_MMC/MMC/armB_b/SubModule3/cell voltage ==
  SOC : Inport
  Constant : Constant  Value=3
  Gain : Gain  Gain=1.2
  Sum : Sum  Inputs=|++
  V : Outport
  wires:
  Sum/1 -> V/1
  SOC/1 -> Gain/1
  Gain/1 -> Sum/2
  Constant/1 -> Sum/1

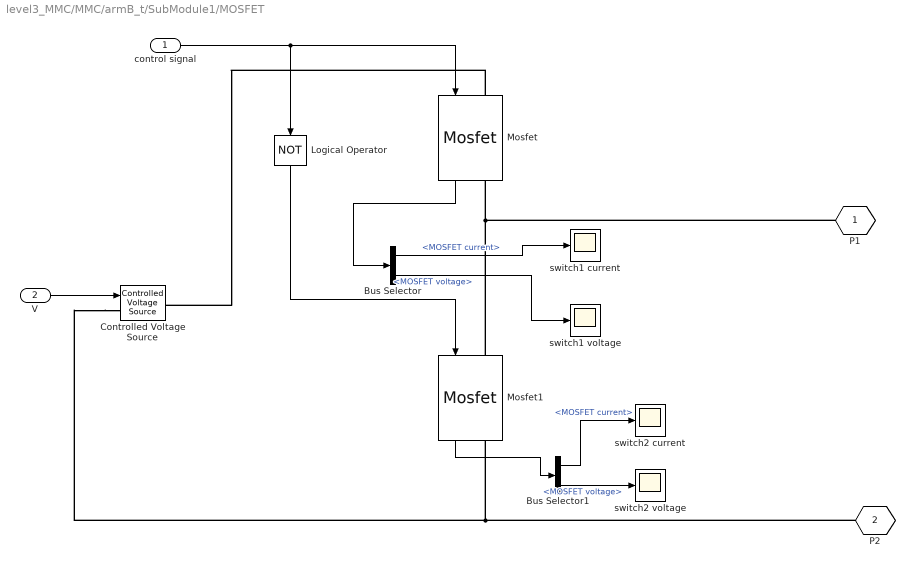
== system level3_MMC/MMC/armB_t/SubModule1/MOSFET ==
  control signal : Inport
  V : Inport  Port=2
  Bus Selector : BusSelector  OutputSignals=MOSFET current,MOSFET voltage
  Bus Selector1 : BusSelector  OutputSignals=MOSFET current,MOSFET voltage
  Controlled Voltage Source : powerlib/Electrical Sources/Controlled Voltage Source  Initialize=on  Source_Type=AC  Amplitude=0  Phase=0  Frequency=0  Measurements=None
  Logical Operator : Logic  Operator=NOT  AllPortsSameDT=off  OutDataTypeStr=boolean
  Mosfet : powerlib/Power Electronics/Mosfet  Ron=0.0005  Lon=0  Rd=0.01  Vfd=0  IC=0  Rs=1e5  Cs=inf  Measurements=on
  Mosfet1 : powerlib/Power Electronics/Mosfet  Ron=0.0005  Lon=0  Rd=0.01  Vfd=0  IC=0  Rs=1e5  Cs=inf  Measurements=on
  switch1 current : Scope
  switch1 voltage : Scope
  switch2 current : Scope
  switch2 voltage : Scope
  P1 : PMIOPort  Tag=PMCPort  Port=1  Side=Right
  P2 : PMIOPort  Tag=PMCPort  Port=2  Side=Right
  wires:
  control signal/1 -> Logical Operator/1, Mosfet/1
  Mosfet/1 -> Bus Selector/1
  V/1 -> Controlled Voltage Source/1
  Bus Selector/1 -> switch1 current/1  "<MOSFET current>"
  Bus Selector/2 -> switch1 voltage/1  "<MOSFET voltage>"
  Bus Selector1/1 -> switch2 current/1  "<MOSFET current>"
  Bus Selector1/2 -> switch2 voltage/1  "<MOSFET voltage>"
  Logical Operator/1 -> Mosfet1/1
  Mosfet1/1 -> Bus Selector1/1
  connections:
  Controlled Voltage Source/LConn1 -- Mosfet1/RConn1 -- P2/RConn1
  Mosfet1/LConn1 -- Mosfet/RConn1 -- P1/RConn1
  Mosfet/LConn1 -- Controlled Voltage Source/RConn1

== system level3_MMC/MMC/armB_t/SubModule1/cell voltage ==
  SOC : Inport
  Constant : Constant  Value=3
  Gain : Gain  Gain=1.2
  Sum : Sum  Inputs=|++
  V : Outport
  wires:
  Sum/1 -> V/1
  SOC/1 -> Gain/1
  Gain/1 -> Sum/2
  Constant/1 -> Sum/1

== system level3_MMC/MMC/armB_t/SubModule2/MOSFET ==
  control signal : Inport
  V : Inport  Port=2
  Bus Selector : BusSelector  OutputSignals=MOSFET current,MOSFET voltage
  Bus Selector1 : BusSelector  OutputSignals=MOSFET current,MOSFET voltage
  Controlled Voltage Source : powerlib/Electrical Sources/Controlled Voltage Source  Initialize=on  Source_Type=AC  Amplitude=0  Phase=0  Frequency=0  Measurements=None
  Logical Operator : Logic  Operator=NOT  AllPortsSameDT=off  OutDataTypeStr=boolean
  Mosfet : powerlib/Power Electronics/Mosfet  Ron=0.0005  Lon=0  Rd=0.01  Vfd=0  IC=0  Rs=1e5  Cs=inf  Measurements=on
  Mosfet1 : powerlib/Power Electronics/Mosfet  Ron=0.0005  Lon=0  Rd=0.01  Vfd=0  IC=0  Rs=1e5  Cs=inf  Measurements=on
  switch1 current : Scope
  switch1 voltage : Scope
  switch2 current : Scope
  switch2 voltage : Scope
  P1 : PMIOPort  Tag=PMCPort  Port=1  Side=Right
  P2 : PMIOPort  Tag=PMCPort  Port=2  Side=Right
  wires:
  control signal/1 -> Logical Operator/1, Mosfet/1
  Mosfet/1 -> Bus Selector/1
  V/1 -> Controlled Voltage Source/1
  Bus Selector/1 -> switch1 current/1  "<MOSFET current>"
  Bus Selector/2 -> switch1 voltage/1  "<MOSFET voltage>"
  Bus Selector1/1 -> switch2 current/1  "<MOSFET current>"
  Bus Selector1/2 -> switch2 voltage/1  "<MOSFET voltage>"
  Logical Operator/1 -> Mosfet1/1
  Mosfet1/1 -> Bus Selector1/1
  connections:
  Controlled Voltage Source/LConn1 -- Mosfet1/RConn1 -- P2/RConn1
  Mosfet1/LConn1 -- Mosfet/RConn1 -- P1/RConn1
  Mosfet/LConn1 -- Controlled Voltage Source/RConn1

== system level3_MMC/MMC/armB_t/SubModule2/cell voltage ==
  SOC : Inport
  Constant : Constant  Value=3
  Gain : Gain  Gain=1.2
  Sum : Sum  Inputs=|++
  V : Outport
  wires:
  Sum/1 -> V/1
  SOC/1 -> Gain/1
  Gain/1 -> Sum/2
  Constant/1 -> Sum/1

== system level3_MMC/MMC/armB_t/SubModule3/MOSFET ==
  control signal : Inport
  V : Inport  Port=2
  Bus Selector : BusSelector  OutputSignals=MOSFET current,MOSFET voltage
  Bus Selector1 : BusSelector  OutputSignals=MOSFET current,MOSFET voltage
  Controlled Voltage Source : powerlib/Electrical Sources/Controlled Voltage Source  Initialize=on  Source_Type=AC  Amplitude=0  Phase=0  Frequency=0  Measurements=None
  Logical Operator : Logic  Operator=NOT  AllPortsSameDT=off  OutDataTypeStr=boolean
  Mosfet : powerlib/Power Electronics/Mosfet  Ron=0.0005  Lon=0  Rd=0.01  Vfd=0  IC=0  Rs=1e5  Cs=inf  Measurements=on
  Mosfet1 : powerlib/Power Electronics/Mosfet  Ron=0.0005  Lon=0  Rd=0.01  Vfd=0  IC=0  Rs=1e5  Cs=inf  Measurements=on
  switch1 current : Scope
  switch1 voltage : Scope
  switch2 current : Scope
  switch2 voltage : Scope
  P1 : PMIOPort  Tag=PMCPort  Port=1  Side=Right
  P2 : PMIOPort  Tag=PMCPort  Port=2  Side=Right
  wires:
  control signal/1 -> Logical Operator/1, Mosfet/1
  Mosfet/1 -> Bus Selector/1
  V/1 -> Controlled Voltage Source/1
  Bus Selector/1 -> switch1 current/1  "<MOSFET current>"
  Bus Selector/2 -> switch1 voltage/1  "<MOSFET voltage>"
  Bus Selector1/1 -> switch2 current/1  "<MOSFET current>"
  Bus Selector1/2 -> switch2 voltage/1  "<MOSFET voltage>"
  Logical Operator/1 -> Mosfet1/1
  Mosfet1/1 -> Bus Selector1/1
  connections:
  Controlled Voltage Source/LConn1 -- Mosfet1/RConn1 -- P2/RConn1
  Mosfet1/LConn1 -- Mosfet/RConn1 -- P1/RConn1
  Mosfet/LConn1 -- Controlled Voltage Source/RConn1

== system level3_MMC/MMC/armB_t/SubModule3/cell voltage ==
  SOC : Inport
  Constant : Constant  Value=3
  Gain : Gain  Gain=1.2
  Sum : Sum  Inputs=|++
  V : Outport
  wires:
  Sum/1 -> V/1
  SOC/1 -> Gain/1
  Gain/1 -> Sum/2
  Constant/1 -> Sum/1

== system level3_MMC/MMC/armC_b/SubModule1/MOSFET ==
  control signal : Inport
  V : Inport  Port=2
  Bus Selector : BusSelector  OutputSignals=MOSFET current,MOSFET voltage
  Bus Selector1 : BusSelector  OutputSignals=MOSFET current,MOSFET voltage
  Controlled Voltage Source : powerlib/Electrical Sources/Controlled Voltage Source  Initialize=on  Source_Type=AC  Amplitude=0  Phase=0  Frequency=0  Measurements=None
  Logical Operator : Logic  Operator=NOT  AllPortsSameDT=off  OutDataTypeStr=boolean
  Mosfet : powerlib/Power Electronics/Mosfet  Ron=0.0005  Lon=0  Rd=0.01  Vfd=0  IC=0  Rs=1e5  Cs=inf  Measurements=on
  Mosfet1 : powerlib/Power Electronics/Mosfet  Ron=0.0005  Lon=0  Rd=0.01  Vfd=0  IC=0  Rs=1e5  Cs=inf  Measurements=on
  switch1 current : Scope
  switch1 voltage : Scope
  switch2 current : Scope
  switch2 voltage : Scope
  P1 : PMIOPort  Tag=PMCPort  Port=1  Side=Right
  P2 : PMIOPort  Tag=PMCPort  Port=2  Side=Right
  wires:
  control signal/1 -> Logical Operator/1, Mosfet/1
  Mosfet/1 -> Bus Selector/1
  V/1 -> Controlled Voltage Source/1
  Bus Selector/1 -> switch1 current/1  "<MOSFET current>"
  Bus Selector/2 -> switch1 voltage/1  "<MOSFET voltage>"
  Bus Selector1/1 -> switch2 current/1  "<MOSFET current>"
  Bus Selector1/2 -> switch2 voltage/1  "<MOSFET voltage>"
  Logical Operator/1 -> Mosfet1/1
  Mosfet1/1 -> Bus Selector1/1
  connections:
  Controlled Voltage Source/LConn1 -- Mosfet1/RConn1 -- P2/RConn1
  Mosfet1/LConn1 -- Mosfet/RConn1 -- P1/RConn1
  Mosfet/LConn1 -- Controlled Voltage Source/RConn1

== system level3_MMC/MMC/armC_b/SubModule1/cell voltage ==
  SOC : Inport
  Constant : Constant  Value=3
  Gain : Gain  Gain=1.2
  Sum : Sum  Inputs=|++
  V : Outport
  wires:
  Sum/1 -> V/1
  SOC/1 -> Gain/1
  Gain/1 -> Sum/2
  Constant/1 -> Sum/1

== system level3_MMC/MMC/armC_b/SubModule2/MOSFET ==
  control signal : Inport
  V : Inport  Port=2
  Bus Selector : BusSelector  OutputSignals=MOSFET current,MOSFET voltage
  Bus Selector1 : BusSelector  OutputSignals=MOSFET current,MOSFET voltage
  Controlled Voltage Source : powerlib/Electrical Sources/Controlled Voltage Source  Initialize=on  Source_Type=AC  Amplitude=0  Phase=0  Frequency=0  Measurements=None
  Logical Operator : Logic  Operator=NOT  AllPortsSameDT=off  OutDataTypeStr=boolean
  Mosfet : powerlib/Power Electronics/Mosfet  Ron=0.0005  Lon=0  Rd=0.01  Vfd=0  IC=0  Rs=1e5  Cs=inf  Measurements=on
  Mosfet1 : powerlib/Power Electronics/Mosfet  Ron=0.0005  Lon=0  Rd=0.01  Vfd=0  IC=0  Rs=1e5  Cs=inf  Measurements=on
  switch1 current : Scope
  switch1 voltage : Scope
  switch2 current : Scope
  switch2 voltage : Scope
  P1 : PMIOPort  Tag=PMCPort  Port=1  Side=Right
  P2 : PMIOPort  Tag=PMCPort  Port=2  Side=Right
  wires:
  control signal/1 -> Logical Operator/1, Mosfet/1
  Mosfet/1 -> Bus Selector/1
  V/1 -> Controlled Voltage Source/1
  Bus Selector/1 -> switch1 current/1  "<MOSFET current>"
  Bus Selector/2 -> switch1 voltage/1  "<MOSFET voltage>"
  Bus Selector1/1 -> switch2 current/1  "<MOSFET current>"
  Bus Selector1/2 -> switch2 voltage/1  "<MOSFET voltage>"
  Logical Operator/1 -> Mosfet1/1
  Mosfet1/1 -> Bus Selector1/1
  connections:
  Controlled Voltage Source/LConn1 -- Mosfet1/RConn1 -- P2/RConn1
  Mosfet1/LConn1 -- Mosfet/RConn1 -- P1/RConn1
  Mosfet/LConn1 -- Controlled Voltage Source/RConn1

== system level3_MMC/MMC/armC_b/SubModule2/cell voltage ==
  SOC : Inport
  Constant : Constant  Value=3
  Gain : Gain  Gain=1.2
  Sum : Sum  Inputs=|++
  V : Outport
  wires:
  Sum/1 -> V/1
  SOC/1 -> Gain/1
  Gain/1 -> Sum/2
  Constant/1 -> Sum/1

== system level3_MMC/MMC/armC_b/SubModule3/MOSFET ==
  control signal : Inport
  V : Inport  Port=2
  Bus Selector : BusSelector  OutputSignals=MOSFET current,MOSFET voltage
  Bus Selector1 : BusSelector  OutputSignals=MOSFET current,MOSFET voltage
  Controlled Voltage Source : powerlib/Electrical Sources/Controlled Voltage Source  Initialize=on  Source_Type=AC  Amplitude=0  Phase=0  Frequency=0  Measurements=None
  Logical Operator : Logic  Operator=NOT  AllPortsSameDT=off  OutDataTypeStr=boolean
  Mosfet : powerlib/Power Electronics/Mosfet  Ron=0.0005  Lon=0  Rd=0.01  Vfd=0  IC=0  Rs=1e5  Cs=inf  Measurements=on
  Mosfet1 : powerlib/Power Electronics/Mosfet  Ron=0.0005  Lon=0  Rd=0.01  Vfd=0  IC=0  Rs=1e5  Cs=inf  Measurements=on
  switch1 current : Scope
  switch1 voltage : Scope
  switch2 current : Scope
  switch2 voltage : Scope
  P1 : PMIOPort  Tag=PMCPort  Port=1  Side=Right
  P2 : PMIOPort  Tag=PMCPort  Port=2  Side=Right
  wires:
  control signal/1 -> Logical Operator/1, Mosfet/1
  Mosfet/1 -> Bus Selector/1
  V/1 -> Controlled Voltage Source/1
  Bus Selector/1 -> switch1 current/1  "<MOSFET current>"
  Bus Selector/2 -> switch1 voltage/1  "<MOSFET voltage>"
  Bus Selector1/1 -> switch2 current/1  "<MOSFET current>"
  Bus Selector1/2 -> switch2 voltage/1  "<MOSFET voltage>"
  Logical Operator/1 -> Mosfet1/1
  Mosfet1/1 -> Bus Selector1/1
  connections:
  Controlled Voltage Source/LConn1 -- Mosfet1/RConn1 -- P2/RConn1
  Mosfet1/LConn1 -- Mosfet/RConn1 -- P1/RConn1
  Mosfet/LConn1 -- Controlled Voltage Source/RConn1

== system level3_MMC/MMC/armC_b/SubModule3/cell voltage ==
  SOC : Inport
  Constant : Constant  Value=3
  Gain : Gain  Gain=1.2
  Sum : Sum  Inputs=|++
  V : Outport
  wires:
  Sum/1 -> V/1
  SOC/1 -> Gain/1
  Gain/1 -> Sum/2
  Constant/1 -> Sum/1

== system level3_MMC/MMC/armC_t/SubModule1/MOSFET ==
  control signal : Inport
  V : Inport  Port=2
  Bus Selector : BusSelector  OutputSignals=MOSFET current,MOSFET voltage
  Bus Selector1 : BusSelector  OutputSignals=MOSFET current,MOSFET voltage
  Controlled Voltage Source : powerlib/Electrical Sources/Controlled Voltage Source  Initialize=on  Source_Type=AC  Amplitude=0  Phase=0  Frequency=0  Measurements=None
  Logical Operator : Logic  Operator=NOT  AllPortsSameDT=off  OutDataTypeStr=boolean
  Mosfet : powerlib/Power Electronics/Mosfet  Ron=0.0005  Lon=0  Rd=0.01  Vfd=0  IC=0  Rs=1e5  Cs=inf  Measurements=on
  Mosfet1 : powerlib/Power Electronics/Mosfet  Ron=0.0005  Lon=0  Rd=0.01  Vfd=0  IC=0  Rs=1e5  Cs=inf  Measurements=on
  switch1 current : Scope
  switch1 voltage : Scope
  switch2 current : Scope
  switch2 voltage : Scope
  P1 : PMIOPort  Tag=PMCPort  Port=1  Side=Right
  P2 : PMIOPort  Tag=PMCPort  Port=2  Side=Right
  wires:
  control signal/1 -> Logical Operator/1, Mosfet/1
  Mosfet/1 -> Bus Selector/1
  V/1 -> Controlled Voltage Source/1
  Bus Selector/1 -> switch1 current/1  "<MOSFET current>"
  Bus Selector/2 -> switch1 voltage/1  "<MOSFET voltage>"
  Bus Selector1/1 -> switch2 current/1  "<MOSFET current>"
  Bus Selector1/2 -> switch2 voltage/1  "<MOSFET voltage>"
  Logical Operator/1 -> Mosfet1/1
  Mosfet1/1 -> Bus Selector1/1
  connections:
  Controlled Voltage Source/LConn1 -- Mosfet1/RConn1 -- P2/RConn1
  Mosfet1/LConn1 -- Mosfet/RConn1 -- P1/RConn1
  Mosfet/LConn1 -- Controlled Voltage Source/RConn1

== system level3_MMC/MMC/armC_t/SubModule1/cell voltage ==
  SOC : Inport
  Constant : Constant  Value=3
  Gain : Gain  Gain=1.2
  Sum : Sum  Inputs=|++
  V : Outport
  wires:
  Sum/1 -> V/1
  SOC/1 -> Gain/1
  Gain/1 -> Sum/2
  Constant/1 -> Sum/1

== system level3_MMC/MMC/armC_t/SubModule2/MOSFET ==
  control signal : Inport
  V : Inport  Port=2
  Bus Selector : BusSelector  OutputSignals=MOSFET current,MOSFET voltage
  Bus Selector1 : BusSelector  OutputSignals=MOSFET current,MOSFET voltage
  Controlled Voltage Source : powerlib/Electrical Sources/Controlled Voltage Source  Initialize=on  Source_Type=AC  Amplitude=0  Phase=0  Frequency=0  Measurements=None
  Logical Operator : Logic  Operator=NOT  AllPortsSameDT=off  OutDataTypeStr=boolean
  Mosfet : powerlib/Power Electronics/Mosfet  Ron=0.0005  Lon=0  Rd=0.01  Vfd=0  IC=0  Rs=1e5  Cs=inf  Measurements=on
  Mosfet1 : powerlib/Power Electronics/Mosfet  Ron=0.0005  Lon=0  Rd=0.01  Vfd=0  IC=0  Rs=1e5  Cs=inf  Measurements=on
  switch1 current : Scope
  switch1 voltage : Scope
  switch2 current : Scope
  switch2 voltage : Scope
  P1 : PMIOPort  Tag=PMCPort  Port=1  Side=Right
  P2 : PMIOPort  Tag=PMCPort  Port=2  Side=Right
  wires:
  control signal/1 -> Logical Operator/1, Mosfet/1
  Mosfet/1 -> Bus Selector/1
  V/1 -> Controlled Voltage Source/1
  Bus Selector/1 -> switch1 current/1  "<MOSFET current>"
  Bus Selector/2 -> switch1 voltage/1  "<MOSFET voltage>"
  Bus Selector1/1 -> switch2 current/1  "<MOSFET current>"
  Bus Selector1/2 -> switch2 voltage/1  "<MOSFET voltage>"
  Logical Operator/1 -> Mosfet1/1
  Mosfet1/1 -> Bus Selector1/1
  connections:
  Controlled Voltage Source/LConn1 -- Mosfet1/RConn1 -- P2/RConn1
  Mosfet1/LConn1 -- Mosfet/RConn1 -- P1/RConn1
  Mosfet/LConn1 -- Controlled Voltage Source/RConn1

== system level3_MMC/MMC/armC_t/SubModule2/cell voltage ==
  SOC : Inport
  Constant : Constant  Value=3
  Gain : Gain  Gain=1.2
  Sum : Sum  Inputs=|++
  V : Outport
  wires:
  Sum/1 -> V/1
  SOC/1 -> Gain/1
  Gain/1 -> Sum/2
  Constant/1 -> Sum/1

== system level3_MMC/MMC/armC_t/SubModule3/MOSFET ==
  control signal : Inport
  V : Inport  Port=2
  Bus Selector : BusSelector  OutputSignals=MOSFET current,MOSFET voltage
  Bus Selector1 : BusSelector  OutputSignals=MOSFET current,MOSFET voltage
  Controlled Voltage Source : powerlib/Electrical Sources/Controlled Voltage Source  Initialize=on  Source_Type=AC  Amplitude=0  Phase=0  Frequency=0  Measurements=None
  Logical Operator : Logic  Operator=NOT  AllPortsSameDT=off  OutDataTypeStr=boolean
  Mosfet : powerlib/Power Electronics/Mosfet  Ron=0.0005  Lon=0  Rd=0.01  Vfd=0  IC=0  Rs=1e5  Cs=inf  Measurements=on
  Mosfet1 : powerlib/Power Electronics/Mosfet  Ron=0.0005  Lon=0  Rd=0.01  Vfd=0  IC=0  Rs=1e5  Cs=inf  Measurements=on
  switch1 current : Scope
  switch1 voltage : Scope
  switch2 current : Scope
  switch2 voltage : Scope
  P1 : PMIOPort  Tag=PMCPort  Port=1  Side=Right
  P2 : PMIOPort  Tag=PMCPort  Port=2  Side=Right
  wires:
  control signal/1 -> Logical Operator/1, Mosfet/1
  Mosfet/1 -> Bus Selector/1
  V/1 -> Controlled Voltage Source/1
  Bus Selector/1 -> switch1 current/1  "<MOSFET current>"
  Bus Selector/2 -> switch1 voltage/1  "<MOSFET voltage>"
  Bus Selector1/1 -> switch2 current/1  "<MOSFET current>"
  Bus Selector1/2 -> switch2 voltage/1  "<MOSFET voltage>"
  Logical Operator/1 -> Mosfet1/1
  Mosfet1/1 -> Bus Selector1/1
  connections:
  Controlled Voltage Source/LConn1 -- Mosfet1/RConn1 -- P2/RConn1
  Mosfet1/LConn1 -- Mosfet/RConn1 -- P1/RConn1
  Mosfet/LConn1 -- Controlled Voltage Source/RConn1

== system level3_MMC/MMC/armC_t/SubModule3/cell voltage ==
  SOC : Inport
  Constant : Constant  Value=3
  Gain : Gain  Gain=1.2
  Sum : Sum  Inputs=|++
  V : Outport
  wires:
  Sum/1 -> V/1
  SOC/1 -> Gain/1
  Gain/1 -> Sum/2
  Constant/1 -> Sum/1
